simulink model "Spike_Generator_matt"  (R2019b)
settings: Solver=VariableStepAuto  StartTime=0.0  StopTime=testtime  RelTol=1e-3
InitFcn:
  | Spike_Generator_Test_Parameters
StopFcn:
  | Verify_Spike_Generator
values from neighbouring files (symbols this model uses):
  Fs = 48e3    (= 48000)    [Spike_Generator_Test_Parameters.m]    (also in modelparameters.m)
  nSites = 4    [Spike_Generator_Test_Parameters.m]
  tabs = 0.6e-3    (= 0.0006)    [Spike_Generator_Test_Parameters.m]
  trel = 0.6e-3    (= 0.0006)    [Spike_Generator_Test_Parameters.m]
libraries: dspsrcs4 x4
(part 1 of 3)
settings Model: NumberOfSteps=50  Creator=mblun  LastModifiedBy=t96f346
settings OptimizationCC: BlockReduction=off  ConditionallyExecuteInputs=off  DefaultParameterBehavior=Inlined
settings DebuggingCC: AlgebraicLoopMsg=error
settings HardwareCC: ProdBitPerPointer=32  ProdBitPerSizeT=32  ProdBitPerPtrDiffT=32  ProdLargestAtomicFloat=None  ProdIntDivRoundTo=Undefined  ProdEndianess=Unspecified  ProdWordSize=32  ProdHWDeviceType=ASIC/FPGA->ASIC/FPGA  TargetBitPerPointer=64  TargetBitPerSizeT=64  TargetBitPerPtrDiffT=64  TargetLongLongMode=on  TargetIntDivRoundTo=Zero  TargetEndianess=LittleEndian  TargetWordSize=64  TargetHWDeviceType=Custom Processor->MATLAB Host Computer  ProdEqTarget=off
settings SFSimCC: CustomCodeUndefinedFunction=UseInterfaceOnly

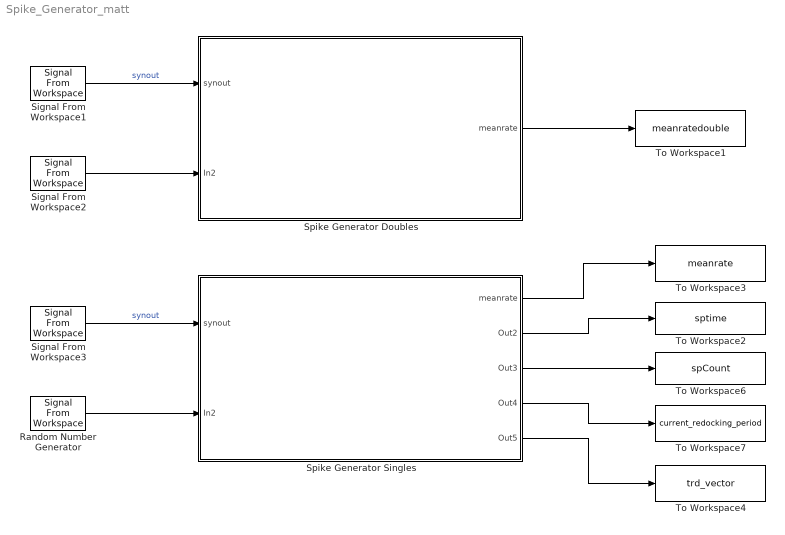
== system Spike_Generator_matt ==
  Random Number Generator : dspsrcs4/Signal From Workspace  X=randNums  Ts=1/Fs  nsamps=1  OutputAfterFinalValue=Setting to zero  ignoreOrWarnInputAndFrameLengths=off  OutputFrames=off
  Signal From Workspace1 : dspsrcs4/Signal From Workspace  X=synoutdouble  Ts=1/Fs  nsamps=1  OutputAfterFinalValue=Setting to zero  ignoreOrWarnInputAndFrameLengths=off  OutputFrames=off
  Signal From Workspace2 : dspsrcs4/Signal From Workspace  X=randNumsdouble  Ts=1/Fs  nsamps=1  OutputAfterFinalValue=Setting to zero  ignoreOrWarnInputAndFrameLengths=off  OutputFrames=off
  Signal From Workspace3 : dspsrcs4/Signal From Workspace  X=synout  Ts=1/Fs  nsamps=1  OutputAfterFinalValue=Setting to zero  ignoreOrWarnInputAndFrameLengths=off  OutputFrames=off
  Spike Generator Doubles : Subsystem
  Spike Generator Singles : Subsystem
  To Workspace1 : ToWorkspace  VariableName=meanratedouble  SampleTime=-1
      settings: Save2DSignal=2-D array (concatenate along first dimension)
  To Workspace2 : ToWorkspace  VariableName=sptime  SampleTime=-1
      settings: Save2DSignal=2-D array (concatenate along first dimension)
  To Workspace3 : ToWorkspace  VariableName=meanrate  SampleTime=-1
      settings: Save2DSignal=2-D array (concatenate along first dimension)
  To Workspace4 : ToWorkspace  VariableName=trd_vector  SampleTime=-1
      settings: Save2DSignal=2-D array (concatenate along first dimension)
  To Workspace6 : ToWorkspace  VariableName=spCount  SampleTime=-1
      settings: Save2DSignal=2-D array (concatenate along first dimension)
  To Workspace7 : ToWorkspace  VariableName=current_redocking_period  SampleTime=-1
      settings: Save2DSignal=2-D array (concatenate along first dimension)
  wires:
  Signal From Workspace1/1 -> Spike Generator Doubles/1(synout)  "synout"
  Signal From Workspace2/1 -> Spike Generator Doubles/2(In2)
  Spike Generator Doubles/1(meanrate) -> To Workspace1/1
  Random Number Generator/1 -> Spike Generator Singles/2(In2)
  Spike Generator Singles/1(meanrate) -> To Workspace3/1
  Signal From Workspace3/1 -> Spike Generator Singles/1(synout)  "synout"
  Spike Generator Singles/2(Out2) -> To Workspace2/1
  Spike Generator Singles/3(Out3) -> To Workspace6/1
  Spike Generator Singles/4(Out4) -> To Workspace7/1
  Spike Generator Singles/5(Out5) -> To Workspace4/1

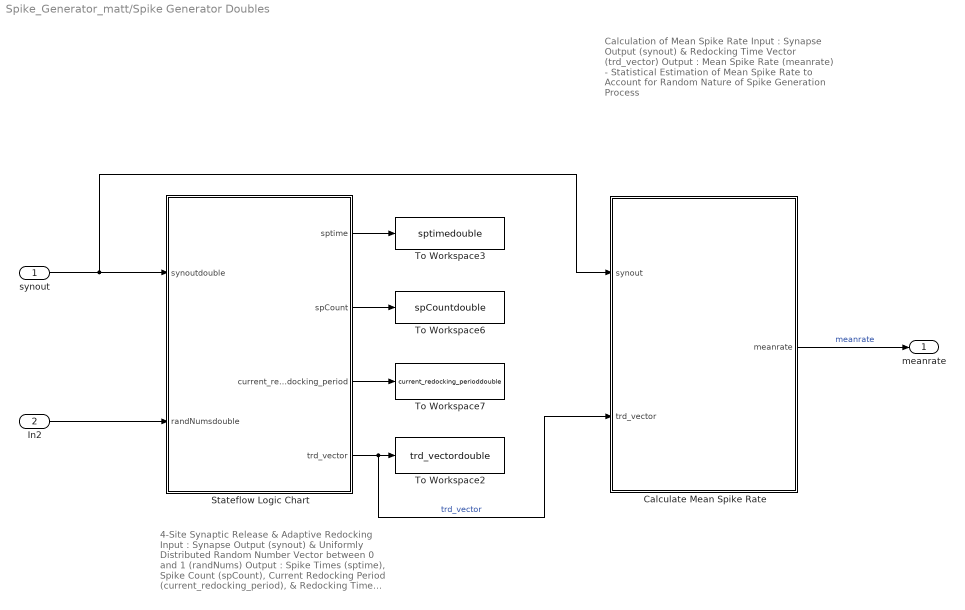
== system Spike_Generator_matt/Spike Generator Doubles ==
  note: 4-Site Synaptic Release & Adaptive Redocking
      |
      | Input : Synapse Output (synout) & Uniformly Distributed Random Number Vector between 0 and 1 (randNums)
      |
      | Output : Spike Times (sptime), Spike Count (spCount), Current Redocking Period (current_redocking_period), & Redocking Time Vector (trd_vector)
      |
      | - Implemented using Stateflow Chart and embedded MATLAB functions
      |
      | - Shows states of synaptic sites during simulation
  note: Calculation of Mean Spike Rate
      |
      | Input : Synapse Output (synout) & Redocking Time Vector (trd_vector)
      |
      | Output : Mean Spike Rate (meanrate)
      |
      | - Statistical Estimation of Mean Spike Rate to Account for Random Nature of Spike Generation Process
  synout : Inport
  In2 : Inport  Port=2
  Calculate Mean Spike Rate : Subsystem
  Stateflow Logic Chart : Stateflow chart  BlockKeywords=__PRM__SERIALIZED__DATA__:Stateflow Chart,Stateflow Diagram  TreatAsAtomicUnit=on
  To Workspace2 : ToWorkspace  VariableName=trd_vectordouble  SampleTime=-1
      settings: Save2DSignal=2-D array (concatenate along first dimension)
  To Workspace3 : ToWorkspace  VariableName=sptimedouble  SampleTime=-1
      settings: Save2DSignal=2-D array (concatenate along first dimension)
  To Workspace6 : ToWorkspace  VariableName=spCountdouble  SampleTime=-1
      settings: Save2DSignal=2-D array (concatenate along first dimension)
  To Workspace7 : ToWorkspace  VariableName=current_redocking_perioddouble  SampleTime=-1
      settings: Save2DSignal=2-D array (concatenate along first dimension)
  meanrate : Outport
  wires:
  Stateflow Logic Chart/2(spCount) -> To Workspace6/1
  In2/1 -> Stateflow Logic Chart/2(randNumsdouble)
  Stateflow Logic Chart/1(sptime) -> To Workspace3/1
  synout/1 -> Calculate Mean Spike Rate/1(synout), Stateflow Logic Chart/1(synoutdouble)
  Stateflow Logic Chart/3(current_redocking_period) -> To Workspace7/1
  Stateflow Logic Chart/4(trd_vector) -> Calculate Mean Spike Rate/2(trd_vector), To Workspace2/1  "trd_vector"
  Calculate Mean Spike Rate/1(meanrate) -> meanrate/1  "meanrate"

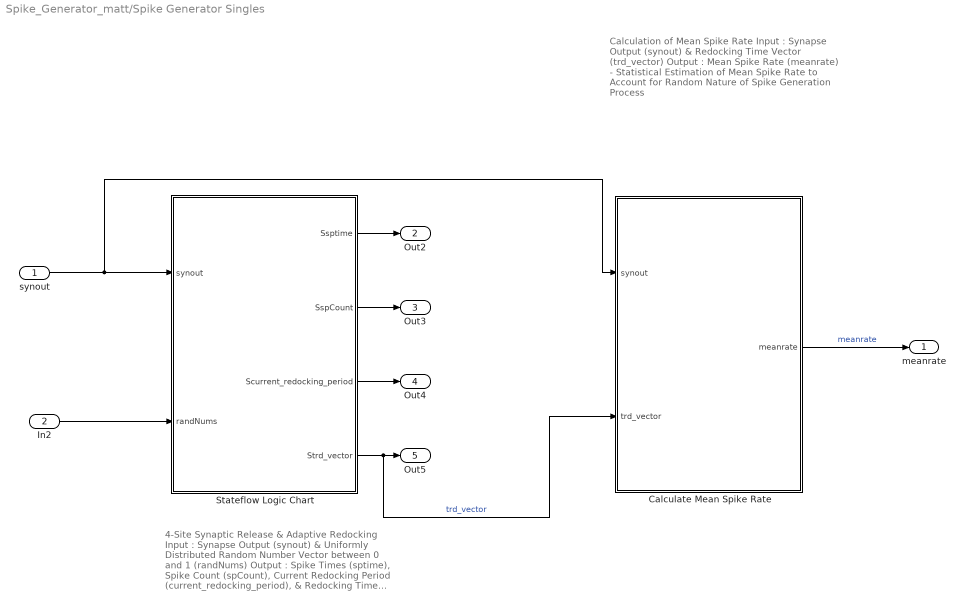
== system Spike_Generator_matt/Spike Generator Singles ==
  note: 4-Site Synaptic Release & Adaptive Redocking
      |
      | Input : Synapse Output (synout) & Uniformly Distributed Random Number Vector between 0 and 1 (randNums)
      |
      | Output : Spike Times (sptime), Spike Count (spCount), Current Redocking Period (current_redocking_period), & Redocking Time Vector (trd_vector)
      |
      | - Implemented using Stateflow Chart and embedded MATLAB functions
      |
      | - Shows states of synaptic sites during simulation
  note: Calculation of Mean Spike Rate
      |
      | Input : Synapse Output (synout) & Redocking Time Vector (trd_vector)
      |
      | Output : Mean Spike Rate (meanrate)
      |
      | - Statistical Estimation of Mean Spike Rate to Account for Random Nature of Spike Generation Process
  synout : Inport
  In2 : Inport  Port=2
  Calculate Mean Spike Rate : Subsystem
  Stateflow Logic Chart : Stateflow chart  BlockKeywords=__PRM__SERIALIZED__DATA__:Stateflow Chart,Stateflow Diagram  TreatAsAtomicUnit=on
  meanrate : Outport
  Out2 : Outport  Port=2
  Out3 : Outport  Port=3
  Out4 : Outport  Port=4
  Out5 : Outport  Port=5
  wires:
  Stateflow Logic Chart/3(Scurrent_redocking_period) -> Out4/1
  synout/1 -> Stateflow Logic Chart/1(synout), Calculate Mean Spike Rate/1(synout)
  Stateflow Logic Chart/4(Strd_vector) -> Out5/1, Calculate Mean Spike Rate/2(trd_vector)  "trd_vector"
  Stateflow Logic Chart/2(SspCount) -> Out3/1
  Stateflow Logic Chart/1(Ssptime) -> Out2/1
  Calculate Mean Spike Rate/1(meanrate) -> meanrate/1  "meanrate"
  In2/1 -> Stateflow Logic Chart/2(randNums)

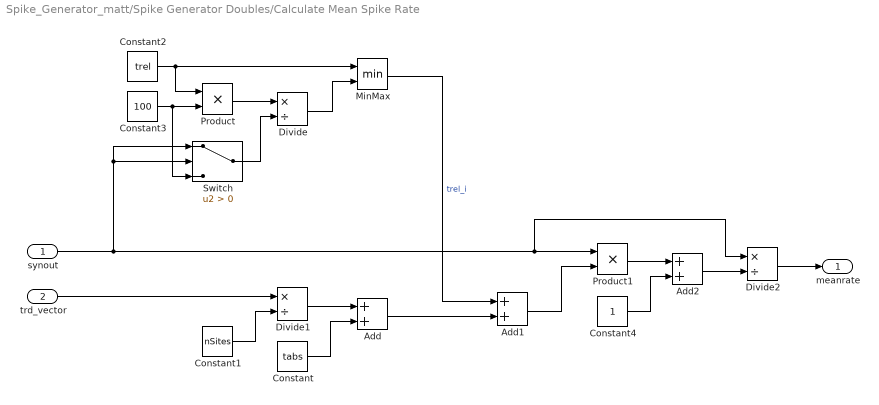
== system Spike_Generator_matt/Spike Generator Doubles/Calculate Mean Spike Rate ==
  synout : Inport
  trd_vector : Inport  Port=2
  Add : Sum
  Add1 : Sum
  Add2 : Sum
  Constant : Constant  Value=tabs  SampleTime=-1
  Constant1 : Constant  Value=nSites  SampleTime=-1
  Constant2 : Constant  Value=trel  SampleTime=-1
  Constant3 : Constant  Value=100  SampleTime=-1
  Constant4 : Constant  SampleTime=-1
  Divide : Product  Inputs=*/  SaturateOnIntegerOverflow=on  RndMeth=Zero
  Divide1 : Product  Inputs=*/  SaturateOnIntegerOverflow=on  RndMeth=Zero
  Divide2 : Product  Inputs=*/  SaturateOnIntegerOverflow=on  RndMeth=Zero
  MinMax : MinMax  Inputs=2
  Product : Product
  Product1 : Product
  Switch : Switch  Criteria=u2 > Threshold
  meanrate : Outport  VectorParamsAs1DForOutWhenUnconnected=off
  wires:
  synout/1 -> Switch/1, Switch/2, Divide2/1, Product1/1
  trd_vector/1 -> Divide1/1
  Constant2/1 -> MinMax/1, Product/1
  Constant3/1 -> Switch/3, Product/2
  Product/1 -> Divide/1
  Divide/1 -> MinMax/2
  MinMax/1 -> Add1/1  "trel_i"
  Constant1/1 -> Divide1/2
  Divide1/1 -> Add/1
  Constant/1 -> Add/2
  Add/1 -> Add1/2
  Constant4/1 -> Add2/2
  Add1/1 -> Product1/2
  Product1/1 -> Add2/1
  Add2/1 -> Divide2/2
  Divide2/1 -> meanrate/1
  Switch/1 -> Divide/2

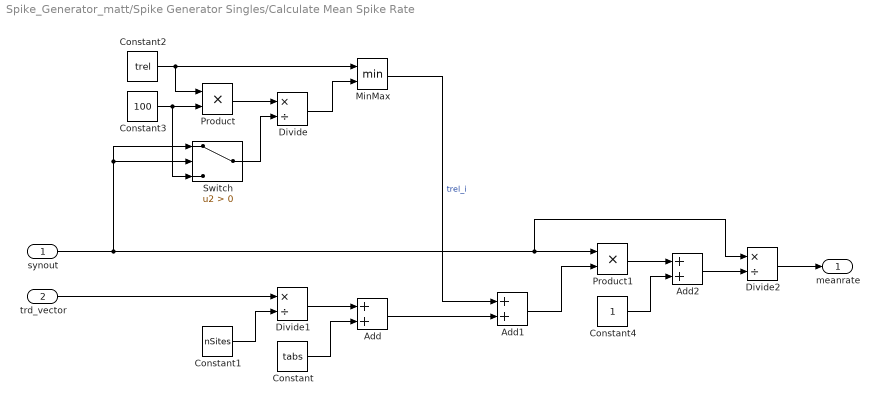
== system Spike_Generator_matt/Spike Generator Singles/Calculate Mean Spike Rate ==
  synout : Inport
  trd_vector : Inport  Port=2
  Add : Sum
  Add1 : Sum
  Add2 : Sum
  Constant : Constant  Value=tabs  OutDataTypeStr=single  SampleTime=-1
  Constant1 : Constant  Value=nSites  OutDataTypeStr=single  SampleTime=-1
  Constant2 : Constant  Value=trel  OutDataTypeStr=single  SampleTime=-1
  Constant3 : Constant  Value=100  OutDataTypeStr=single  SampleTime=-1
  Constant4 : Constant  OutDataTypeStr=single  SampleTime=-1
  Divide : Product  Inputs=*/  SaturateOnIntegerOverflow=on  RndMeth=Zero
  Divide1 : Product  Inputs=*/  SaturateOnIntegerOverflow=on  RndMeth=Zero
  Divide2 : Product  Inputs=*/  SaturateOnIntegerOverflow=on  RndMeth=Zero
  MinMax : MinMax  Inputs=2
  Product : Product
  Product1 : Product
  Switch : Switch  Criteria=u2 > Threshold
  meanrate : Outport  VectorParamsAs1DForOutWhenUnconnected=off
  wires:
  synout/1 -> Switch/1, Switch/2, Divide2/1, Product1/1
  trd_vector/1 -> Divide1/1
  Constant2/1 -> MinMax/1, Product/1
  Constant3/1 -> Switch/3, Product/2
  Product/1 -> Divide/1
  Divide/1 -> MinMax/2
  MinMax/1 -> Add1/1  "trel_i"
  Constant1/1 -> Divide1/2
  Divide1/1 -> Add/1
  Constant/1 -> Add/2
  Add/1 -> Add1/2
  Constant4/1 -> Add2/2
  Add1/1 -> Product1/2
  Product1/1 -> Add2/1
  Add2/1 -> Divide2/2
  Divide2/1 -> meanrate/1
  Switch/1 -> Divide/2
